simulink model "LQR_simulink"  (R2021b)
settings: Solver=VariableStepAuto  StartTime=0.0  StopTime=10  RelTol=1e-3
settings Model: Creator=asus  LastModifiedBy=asus

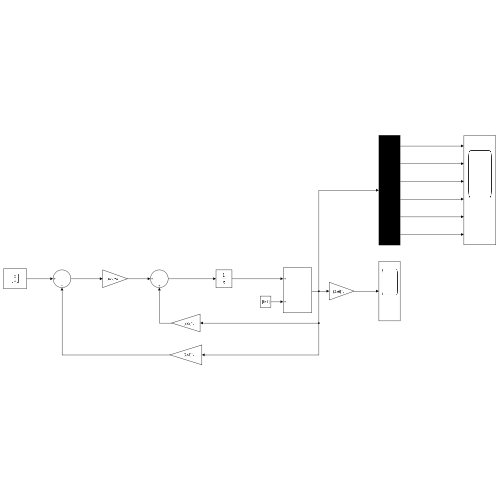
[thumbnail: Simulink's stored preview of the top-level diagram]
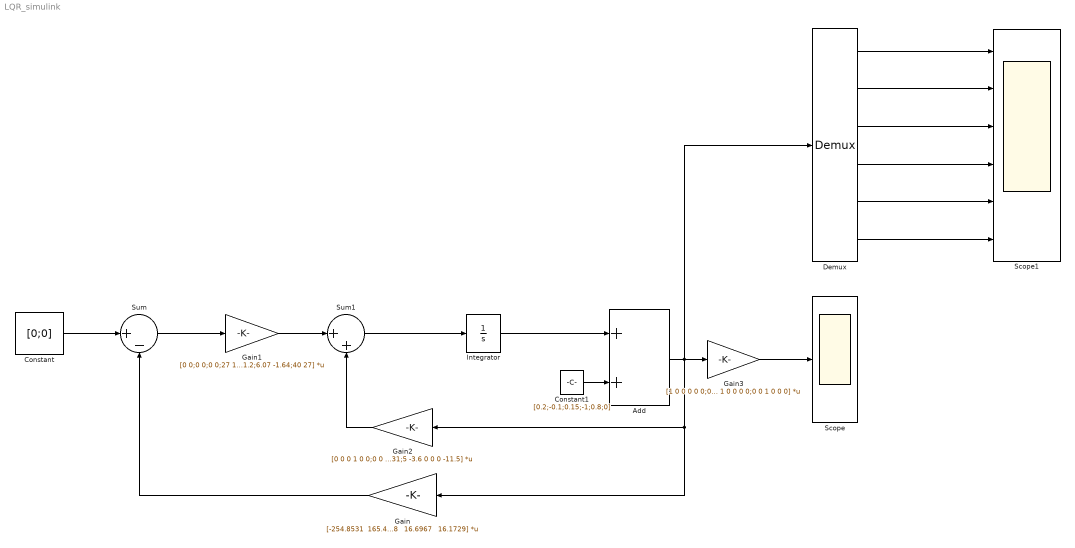
== system LQR_simulink ==
  Add : Sum
  Constant : Constant  Value=[0;0]  VectorParams1D=off
  Constant1 : Constant  Value=[0.2;-0.1;0.15;-1;0.8;0]  VectorParams1D=off
  Demux : Demux  Outputs=6
  Gain : Gain  Gain=|  Multiplication=Matrix(K*u)
      | [-254.8531  165.4206  161.1155  -14.4729   29.5916   15.9109;
      |  -236.3805  135.8063  149.1437  -19.5988   16.6967   16.1729]
  Gain1 : Gain  Gain=[0 0;0 0;0 0;27 11.2;6.07 -1.64;40 27]  Multiplication=Matrix(K*u)
  Gain2 : Gain  Gain=[0 0 0 1 0 0;0 0 0 0 1 0;0 0 0 0 0 1;0 6.5 -10 -15.5 0 0;-22.47 19.4 5.45 -3.48 -4.45 0.31;5 -3.6 0 0 0 -11.5]  Multiplication=Matrix(K*u)
  Gain3 : Gain  Gain=[1 0 0 0 0 0;0 1 0 0 0 0;0 0 1 0 0 0]  Multiplication=Matrix(K*u)
  Integrator : Integrator
  Scope : Scope
  Scope1 : Scope  NumInputPorts=6
  Sum : Sum  Inputs=|+-
  Sum1 : Sum  Inputs=|++
  wires:
  Integrator/1 -> Add/1
  Gain/1 -> Sum/2
  Sum1/1 -> Integrator/1
  Sum/1 -> Gain1/1
  Gain1/1 -> Sum1/1
  Gain2/1 -> Sum1/2
  Constant/1 -> Sum/1
  Gain3/1 -> Scope/1
  Add/1 -> Demux/1, Gain/1, Gain2/1, Gain3/1
  Constant1/1 -> Add/2
  Demux/1 -> Scope1/1
  Demux/2 -> Scope1/2
  Demux/3 -> Scope1/3
  Demux/4 -> Scope1/4
  Demux/5 -> Scope1/5
  Demux/6 -> Scope1/6
